simulink model "slo_constpipe"  (R2015b)
settings: Solver=FixedStepDiscrete  SolverMode=SingleTasking  StartTime=0.0  StopTime=10  RelTol=1e-3
libraries: dspsrcs4 x1, simulink x1
CloseFcn:
  | rtwprivate ssgencode ModelCloseRequest Hysteresis_test1
settings Model: Creator=at-mt  LastModifiedBy=amatsumo
settings DataIOCC: SaveFormat=Array  SignalLoggingSaveFormat=ModelDataLogs  SaveOutput=off  SignalLogging=off  SaveTime=off
settings OptimizationCC: BlockReduction=off  ConditionallyExecuteInputs=off  DefaultParameterBehavior=Inlined  ExpressionDepthLimit=2147483647
settings DebuggingCC: AlgebraicLoopMsg=error  UnderspecifiedInitializationDetection=Classic  MergeDetectMultiDrivingBlocksExec=none  SolverPrmCheckMsg=warning  SingleTaskRateTransMsg=error  FcnCallInpInsideContextMsg=UseLocalSettings  StateNameClashWarn=warning
settings HardwareCC: ProdBitPerPointer=32  ProdLargestAtomicFloat=None  ProdIntDivRoundTo=Undefined  ProdEndianess=Unspecified  ProdWordSize=32  ProdHWDeviceType=ASIC/FPGA->ASIC/FPGA  ProdEqTarget=off
settings GRTTargetCC: GeneratePreprocessorConditionals=Disable all  CombineOutputUpdateFcns=off  GRTInterface=on
settings ConfigComp: CovModelRefEnable=Off  CovSFcnEnable=off

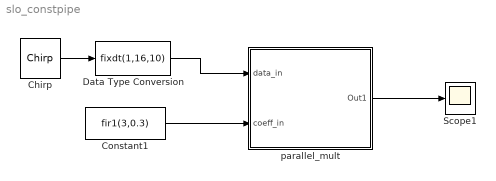
== system slo_constpipe ==
  Chirp : dspsrcs4/Chirp  sweep=Linear  mode=Unidirectional  f0=10  f1=500  t1=10  Tsweep=10  phase=0  Ts=1/1000  spf=1  datatype=Double  OutputFrames=on
  Constant1 : Constant  Value=fir1(3,0.3)  OutDataTypeStr=fixdt(1,16,14)  SampleTime=-1
  Data Type Conversion : DataTypeConversion  OutDataTypeStr=fixdt(1,16,10)
  Scope1 : Scope
  parallel_mult : Subsystem
  wires:
  Chirp/1 -> Data Type Conversion/1
  Data Type Conversion/1 -> parallel_mult/1(data_in)
  Constant1/1 -> parallel_mult/2(coeff_in)
  parallel_mult/1(Out1) -> Scope1/1

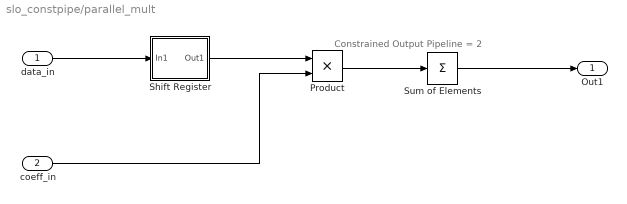
== system slo_constpipe/parallel_mult ==
  note: Constrained Output Pipeline = 2
  data_in : Inport
  coeff_in : Inport  Port=2
  Product : Product  RndMeth=Zero
  Shift Register : Subsystem
  Sum of Elements : Sum  Inputs=+
  Out1 : Outport
  wires:
  data_in/1 -> Shift Register/1(In1)
  Sum of Elements/1 -> Out1/1
  Shift Register/1(Out1) -> Product/1
  coeff_in/1 -> Product/2
  Product/1 -> Sum of Elements/1

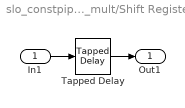
== system slo_constpipe/parallel_mult/Shift Register ==
  In1 : Inport
  Tapped Delay : simulink/Discrete/Tapped Delay  vinit=0.0  samptime=-1  NumDelays=3  DelayOrder=Oldest  includeCurrent=on
  Out1 : Outport
  wires:
  In1/1 -> Tapped Delay/1
  Tapped Delay/1 -> Out1/1
